simulink model "differential_drive_robot2"  (R2024b)
settings: Solver=VariableStepAuto  StartTime=0.0  StopTime=10.0  RelTol=1e-3
libraries: fuzblock x1
settings Model: Creator=aakas  LastModifiedBy=aakas

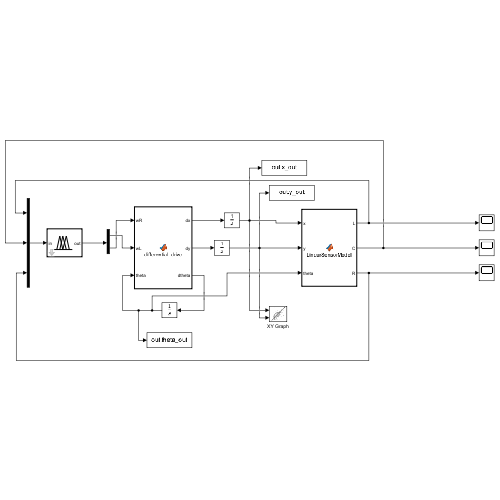
[thumbnail: Simulink's stored preview of the top-level diagram]
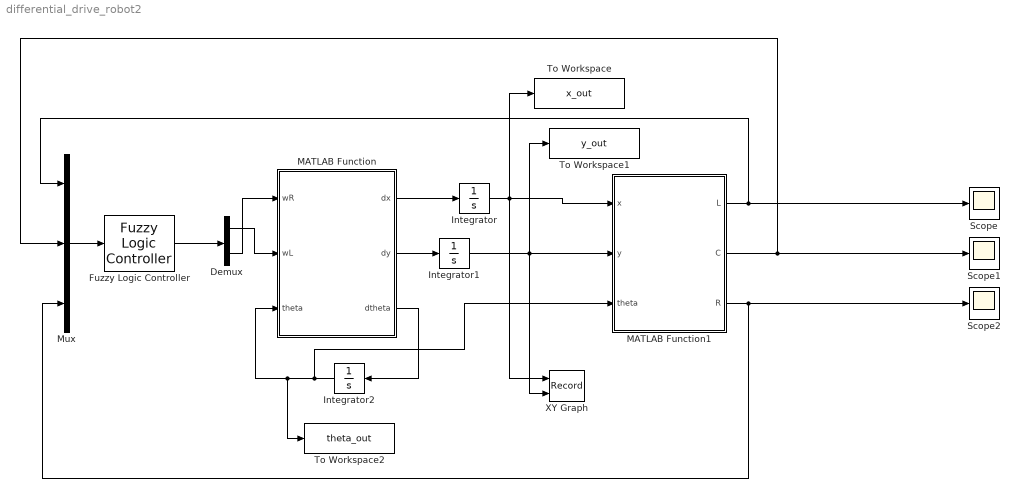
== system differential_drive_robot2 ==
  Demux : Demux  Outputs=2
  Fuzzy Logic Controller : fuzblock/Fuzzy Logic  Controller  FIS="\"line_follower_fuzzy.fis\""  OutputSampleNumber=101  DataType=double  FuzzifiedInputs=off  RuleFiringStrengths=off  RuleOutputs=off  AggregatedOutputs=off  SimulateUsing=Interpreted execution  OutOfRangeInputValueMessage=warning  NoRuleFiredMessage=warning  EmptyOutputFuzzySetMessage=warning
  Integrator : Integrator
  Integrator1 : Integrator
  Integrator2 : Integrator
  MATLAB Function : MATLAB Function  TreatAsAtomicUnit=on
  MATLAB Function1 : MATLAB Function  TreatAsAtomicUnit=on
  Mux : Mux  Inputs=3
  Scope : Scope
  Scope1 : Scope
  Scope2 : Scope
  To Workspace : ToWorkspace  VariableName=x_out  SaveFormat=Structure With Time  SampleTime=-1
  To Workspace1 : ToWorkspace  VariableName=y_out  SaveFormat=Structure With Time  SampleTime=-1
  To Workspace2 : ToWorkspace  VariableName=theta_out  SaveFormat=Structure With Time  SampleTime=-1
  XY Graph : Record  FileSettingsInternal="{\"entries\":[{\"content\":{\"excelSettings\":{\"content\":{},\"type\":\"Streamout.ExcelSettings\"}},\"type\":\"Streamout.FileSettingStorage\",\"uuid\":\"\"}],\"packageUris\":[\"http:\\/\\/schema.mathworks.com\\/mf0\\/streamout_blocks\\/R2020a\"],\"version\":\"1.0\"}"  Layout=[1 1]  SignalsInternal="{\"entries\":[{\"content\":{\"signals\":[{\"content\":{\"blockPath\":[],\"dimensions\":[1],\"domain\":\"\",\"lineColor\":\"#a2142f\",\"plots\":[ 1 ],\"port\":1,\"sid\":[\"\"],\"signalID\":1,\"signalName\":\"Integrator\"},\"type\":\"RecordBlkView.Signal\",\"uuid\":\"\"},{\"content\":{\"blockPath\":[],\"dimensions\":[1],\"domain\":\"\",\"lineColor\":\"#139fff\",\"plots\":[ 1 ],\"port\":2,\"sid\":[\"\"],\"signalID\":2,\"signalName\":\"Integrator1\"},\"type\":\"RecordBlkView.Signal\",\"uuid\":\"\"}]},\"type\":\"RecordBlkView.InputSignals\",\"uuid\":\"\"}],\"packageUris\":[\"http:\\/\\/schema.mathworks.com\\/mf0\\/streamout_blocks\\/R2020a\"],\"version\":\"1.0\"}"  VisualizationBindings="{\"xyplotplugin\":{\"info\":[{\"series\":[{\"bindingParametersList\":[{\"parameter\":\"X-Axis\",\"signalID\":1,\"signalName\":\"Integrator\"},{\"parameter\":\"Y-Axis\",\"signalID\":2,\"signalName\":\"Integrator1\"}],\"seriesID\":0}],\"subplotID\":1}]}}"  CompatibilityTag=XY
  wires:
  MATLAB Function/3(dtheta) -> Integrator2/1
  MATLAB Function/1(dx) -> Integrator/1
  MATLAB Function/2(dy) -> Integrator1/1
  Integrator/1 -> XY Graph/1, To Workspace/1, MATLAB Function1/1(x)
  Mux/1 -> Fuzzy Logic Controller/1
  Fuzzy Logic Controller/1 -> Demux/1
  MATLAB Function1/1(L) -> Mux/1, Scope/1
  MATLAB Function1/2(C) -> Mux/2, Scope1/1
  MATLAB Function1/3(R) -> Scope2/1, Mux/3
  Integrator2/1 -> MATLAB Function1/3(theta), MATLAB Function/3(theta), To Workspace2/1
  Integrator1/1 -> XY Graph/2, To Workspace1/1, MATLAB Function1/2(y)
  Demux/1 -> MATLAB Function/2(wL)
  Demux/2 -> MATLAB Function/1(wR)

== matlab function differential_drive_robot2/MATLAB Function1 ==
  data: x input; L output; C output; R output; y input; theta input
function [L, C, R] = LinearSensorModel(x, y, theta)
    offset = 0.05; % lateral distance between sensors (meters)
    forward = 0.05; % how far in front of the robot they are placed

    % Calculate world coordinates of each sensor
    xC = x + forward * cos(theta);
    yC = y + forward * sin(theta);

    xL = xC - offset * sin(theta);
    yL = yC + offset * cos(theta);

    xR = xC + offset * sin(theta);
    yR = yC - offset * cos(theta);

    % Detect if each sensor is over the black line (y ≈ 0)
    tolerance = 0.01; % line width
    C = abs(yC) < tolerance;
    L = abs(yL) < tolerance;
    R = abs(yR) < tolerance;
end

== matlab function differential_drive_robot2/MATLAB Function ==
  data: wR input; dx output; dy output; dtheta output; wL input; theta input
function [dx, dy, dtheta] = differential_drive(wR, wL, theta)

    r = 0.05; %meters
    L = 0.2; %meters

    v = (r/2) * (wR + wL);
    omega = (r/L) * (wR - wL);

    dx = v * cos(theta);
    dy = omega * sin(theta);
    dtheta = omega;
end
